simulink model "ECU_X_Enumerated_Error_Code_Generator"  (R2022a)
settings: Solver=VariableStepAuto  StartTime=0.0  StopTime=100  RelTol=1e-3
(part 2 of 2)

== system ECU_X_Enumerated_Error_Code_Generator/ECU X Error Processor/If Action Subsystem3/ECU_A_Signal_Error_Flags to Error_Code_Converter/Switch Case Action Subsystem1 ==
  Action Port : ActionPort  ActionPortLabel=case [ 1 ]:
  Constant : Constant  Value=400
  Out1 : Outport  VectorParamsAs1DForOutWhenUnconnected=off
  wires:
  Constant/1 -> Out1/1

== system ECU_X_Enumerated_Error_Code_Generator/ECU X Error Processor/If Action Subsystem3/ECU_A_Signal_Error_Flags to Error_Code_Converter/Switch Case Action Subsystem10 ==
  Action Port : ActionPort  ActionPortLabel=case [ 10 ]:
  Constant : Constant  Value=409
  Out1 : Outport  VectorParamsAs1DForOutWhenUnconnected=off
  wires:
  Constant/1 -> Out1/1

== system ECU_X_Enumerated_Error_Code_Generator/ECU X Error Processor/If Action Subsystem3/ECU_A_Signal_Error_Flags to Error_Code_Converter/Switch Case Action Subsystem11 ==
  Action Port : ActionPort  ActionPortLabel=case [ 11 ]:
  Constant : Constant  Value=500
  Out1 : Outport  VectorParamsAs1DForOutWhenUnconnected=off
  wires:
  Constant/1 -> Out1/1

== system ECU_X_Enumerated_Error_Code_Generator/ECU X Error Processor/If Action Subsystem3/ECU_A_Signal_Error_Flags to Error_Code_Converter/Switch Case Action Subsystem12 ==
  Action Port : ActionPort  ActionPortLabel=case [ 12 ]:
  Constant : Constant  Value=501
  Out1 : Outport  VectorParamsAs1DForOutWhenUnconnected=off
  wires:
  Constant/1 -> Out1/1

== system ECU_X_Enumerated_Error_Code_Generator/ECU X Error Processor/If Action Subsystem3/ECU_A_Signal_Error_Flags to Error_Code_Converter/Switch Case Action Subsystem13 ==
  Action Port : ActionPort  ActionPortLabel=case [ 13 ]:
  Constant : Constant  Value=502
  Out1 : Outport  VectorParamsAs1DForOutWhenUnconnected=off
  wires:
  Constant/1 -> Out1/1

== system ECU_X_Enumerated_Error_Code_Generator/ECU X Error Processor/If Action Subsystem3/ECU_A_Signal_Error_Flags to Error_Code_Converter/Switch Case Action Subsystem14 ==
  Action Port : ActionPort  ActionPortLabel=case [ 14 ]:
  Constant : Constant  Value=503
  Out1 : Outport  VectorParamsAs1DForOutWhenUnconnected=off
  wires:
  Constant/1 -> Out1/1

== system ECU_X_Enumerated_Error_Code_Generator/ECU X Error Processor/If Action Subsystem3/ECU_A_Signal_Error_Flags to Error_Code_Converter/Switch Case Action Subsystem15 ==
  Action Port : ActionPort  ActionPortLabel=case [ 17 ]:
  Constant : Constant  Value=506
  Out1 : Outport  VectorParamsAs1DForOutWhenUnconnected=off
  wires:
  Constant/1 -> Out1/1

== system ECU_X_Enumerated_Error_Code_Generator/ECU X Error Processor/If Action Subsystem3/ECU_A_Signal_Error_Flags to Error_Code_Converter/Switch Case Action Subsystem16 ==
  Action Port : ActionPort  ActionPortLabel=case [ 15 ]:
  Constant : Constant  Value=504
  Out1 : Outport  VectorParamsAs1DForOutWhenUnconnected=off
  wires:
  Constant/1 -> Out1/1

== system ECU_X_Enumerated_Error_Code_Generator/ECU X Error Processor/If Action Subsystem3/ECU_A_Signal_Error_Flags to Error_Code_Converter/Switch Case Action Subsystem17 ==
  Action Port : ActionPort  ActionPortLabel=case [ 16 ]:
  Constant : Constant  Value=505
  Out1 : Outport  VectorParamsAs1DForOutWhenUnconnected=off
  wires:
  Constant/1 -> Out1/1

== system ECU_X_Enumerated_Error_Code_Generator/ECU X Error Processor/If Action Subsystem3/ECU_A_Signal_Error_Flags to Error_Code_Converter/Switch Case Action Subsystem18 ==
  Action Port : ActionPort  ActionPortLabel=case [ 18 ]:
  Constant : Constant  Value=507
  Out1 : Outport  VectorParamsAs1DForOutWhenUnconnected=off
  wires:
  Constant/1 -> Out1/1

== system ECU_X_Enumerated_Error_Code_Generator/ECU X Error Processor/If Action Subsystem3/ECU_A_Signal_Error_Flags to Error_Code_Converter/Switch Case Action Subsystem19 ==
  Action Port : ActionPort  ActionPortLabel=case [ 19 ]:
  Constant : Constant  Value=508
  Out1 : Outport  VectorParamsAs1DForOutWhenUnconnected=off
  wires:
  Constant/1 -> Out1/1

== system ECU_X_Enumerated_Error_Code_Generator/ECU X Error Processor/If Action Subsystem3/ECU_A_Signal_Error_Flags to Error_Code_Converter/Switch Case Action Subsystem2 ==
  Action Port : ActionPort  ActionPortLabel=case [ 2 ]:
  Constant : Constant  Value=401
  Out1 : Outport  VectorParamsAs1DForOutWhenUnconnected=off
  wires:
  Constant/1 -> Out1/1

== system ECU_X_Enumerated_Error_Code_Generator/ECU X Error Processor/If Action Subsystem3/ECU_A_Signal_Error_Flags to Error_Code_Converter/Switch Case Action Subsystem20 ==
  Action Port : ActionPort  ActionPortLabel=case [ 20 ]:
  Constant : Constant  Value=509
  Out1 : Outport  VectorParamsAs1DForOutWhenUnconnected=off
  wires:
  Constant/1 -> Out1/1

== system ECU_X_Enumerated_Error_Code_Generator/ECU X Error Processor/If Action Subsystem3/ECU_A_Signal_Error_Flags to Error_Code_Converter/Switch Case Action Subsystem3 ==
  Action Port : ActionPort  ActionPortLabel=case [ 7 ]:
  Constant : Constant  Value=406
  Out1 : Outport  VectorParamsAs1DForOutWhenUnconnected=off
  wires:
  Constant/1 -> Out1/1

== system ECU_X_Enumerated_Error_Code_Generator/ECU X Error Processor/If Action Subsystem3/ECU_A_Signal_Error_Flags to Error_Code_Converter/Switch Case Action Subsystem4 ==
  Action Port : ActionPort  ActionPortLabel=case [ 3 ]:
  Constant : Constant  Value=402
  Out1 : Outport  VectorParamsAs1DForOutWhenUnconnected=off
  wires:
  Constant/1 -> Out1/1

== system ECU_X_Enumerated_Error_Code_Generator/ECU X Error Processor/If Action Subsystem3/ECU_A_Signal_Error_Flags to Error_Code_Converter/Switch Case Action Subsystem5 ==
  Action Port : ActionPort  ActionPortLabel=case [ 4 ]:
  Constant : Constant  Value=403
  Out1 : Outport  VectorParamsAs1DForOutWhenUnconnected=off
  wires:
  Constant/1 -> Out1/1

== system ECU_X_Enumerated_Error_Code_Generator/ECU X Error Processor/If Action Subsystem3/ECU_A_Signal_Error_Flags to Error_Code_Converter/Switch Case Action Subsystem6 ==
  Action Port : ActionPort  ActionPortLabel=case [ 5 ]:
  Constant : Constant  Value=404
  Out1 : Outport  VectorParamsAs1DForOutWhenUnconnected=off
  wires:
  Constant/1 -> Out1/1

== system ECU_X_Enumerated_Error_Code_Generator/ECU X Error Processor/If Action Subsystem3/ECU_A_Signal_Error_Flags to Error_Code_Converter/Switch Case Action Subsystem7 ==
  Action Port : ActionPort  ActionPortLabel=case [ 6 ]:
  Constant : Constant  Value=405
  Out1 : Outport  VectorParamsAs1DForOutWhenUnconnected=off
  wires:
  Constant/1 -> Out1/1

== system ECU_X_Enumerated_Error_Code_Generator/ECU X Error Processor/If Action Subsystem3/ECU_A_Signal_Error_Flags to Error_Code_Converter/Switch Case Action Subsystem8 ==
  Action Port : ActionPort  ActionPortLabel=case [ 8 ]:
  Constant : Constant  Value=407
  Out1 : Outport  VectorParamsAs1DForOutWhenUnconnected=off
  wires:
  Constant/1 -> Out1/1

== system ECU_X_Enumerated_Error_Code_Generator/ECU X Error Processor/If Action Subsystem3/ECU_A_Signal_Error_Flags to Error_Code_Converter/Switch Case Action Subsystem9 ==
  Action Port : ActionPort  ActionPortLabel=case [ 9 ]:
  Constant : Constant  Value=408
  Out1 : Outport  VectorParamsAs1DForOutWhenUnconnected=off
  wires:
  Constant/1 -> Out1/1

== system ECU_X_Enumerated_Error_Code_Generator/ECU X Error Processor/If Action Subsystem4/ECU_A_Delta_Error_Flags to Error_Code_Converter/Switch Case Action Subsystem1 ==
  Action Port : ActionPort  ActionPortLabel=case [ 1 ]:
  Constant : Constant  Value=600
  Out1 : Outport  VectorParamsAs1DForOutWhenUnconnected=off
  wires:
  Constant/1 -> Out1/1

== system ECU_X_Enumerated_Error_Code_Generator/ECU X Error Processor/If Action Subsystem4/ECU_A_Delta_Error_Flags to Error_Code_Converter/Switch Case Action Subsystem10 ==
  Action Port : ActionPort  ActionPortLabel=case [ 10 ]:
  Constant : Constant  Value=609
  Out1 : Outport  VectorParamsAs1DForOutWhenUnconnected=off
  wires:
  Constant/1 -> Out1/1

== system ECU_X_Enumerated_Error_Code_Generator/ECU X Error Processor/If Action Subsystem4/ECU_A_Delta_Error_Flags to Error_Code_Converter/Switch Case Action Subsystem11 ==
  Action Port : ActionPort  ActionPortLabel=case [ 11 ]:
  Constant : Constant  Value=610
  Out1 : Outport  VectorParamsAs1DForOutWhenUnconnected=off
  wires:
  Constant/1 -> Out1/1

== system ECU_X_Enumerated_Error_Code_Generator/ECU X Error Processor/If Action Subsystem4/ECU_A_Delta_Error_Flags to Error_Code_Converter/Switch Case Action Subsystem12 ==
  Action Port : ActionPort  ActionPortLabel=case [ 12 ]:
  Constant : Constant  Value=611
  Out1 : Outport  VectorParamsAs1DForOutWhenUnconnected=off
  wires:
  Constant/1 -> Out1/1

== system ECU_X_Enumerated_Error_Code_Generator/ECU X Error Processor/If Action Subsystem4/ECU_A_Delta_Error_Flags to Error_Code_Converter/Switch Case Action Subsystem13 ==
  Action Port : ActionPort  ActionPortLabel=case [ 13 ]:
  Constant : Constant  Value=612
  Out1 : Outport  VectorParamsAs1DForOutWhenUnconnected=off
  wires:
  Constant/1 -> Out1/1

== system ECU_X_Enumerated_Error_Code_Generator/ECU X Error Processor/If Action Subsystem4/ECU_A_Delta_Error_Flags to Error_Code_Converter/Switch Case Action Subsystem14 ==
  Action Port : ActionPort  ActionPortLabel=case [ 14 ]:
  Constant : Constant  Value=613
  Out1 : Outport  VectorParamsAs1DForOutWhenUnconnected=off
  wires:
  Constant/1 -> Out1/1

== system ECU_X_Enumerated_Error_Code_Generator/ECU X Error Processor/If Action Subsystem4/ECU_A_Delta_Error_Flags to Error_Code_Converter/Switch Case Action Subsystem15 ==
  Action Port : ActionPort  ActionPortLabel=case [ 17 ]:
  Constant : Constant  Value=700
  Out1 : Outport  VectorParamsAs1DForOutWhenUnconnected=off
  wires:
  Constant/1 -> Out1/1

== system ECU_X_Enumerated_Error_Code_Generator/ECU X Error Processor/If Action Subsystem4/ECU_A_Delta_Error_Flags to Error_Code_Converter/Switch Case Action Subsystem16 ==
  Action Port : ActionPort  ActionPortLabel=case [ 15 ]:
  Constant : Constant  Value=614
  Out1 : Outport  VectorParamsAs1DForOutWhenUnconnected=off
  wires:
  Constant/1 -> Out1/1

== system ECU_X_Enumerated_Error_Code_Generator/ECU X Error Processor/If Action Subsystem4/ECU_A_Delta_Error_Flags to Error_Code_Converter/Switch Case Action Subsystem17 ==
  Action Port : ActionPort  ActionPortLabel=case [ 16 ]:
  Constant : Constant  Value=615
  Out1 : Outport  VectorParamsAs1DForOutWhenUnconnected=off
  wires:
  Constant/1 -> Out1/1

== system ECU_X_Enumerated_Error_Code_Generator/ECU X Error Processor/If Action Subsystem4/ECU_A_Delta_Error_Flags to Error_Code_Converter/Switch Case Action Subsystem18 ==
  Action Port : ActionPort  ActionPortLabel=case [ 18 ]:
  Constant : Constant  Value=701
  Out1 : Outport  VectorParamsAs1DForOutWhenUnconnected=off
  wires:
  Constant/1 -> Out1/1

== system ECU_X_Enumerated_Error_Code_Generator/ECU X Error Processor/If Action Subsystem4/ECU_A_Delta_Error_Flags to Error_Code_Converter/Switch Case Action Subsystem19 ==
  Action Port : ActionPort  ActionPortLabel=case [ 19 ]:
  Constant : Constant  Value=702
  Out1 : Outport  VectorParamsAs1DForOutWhenUnconnected=off
  wires:
  Constant/1 -> Out1/1

== system ECU_X_Enumerated_Error_Code_Generator/ECU X Error Processor/If Action Subsystem4/ECU_A_Delta_Error_Flags to Error_Code_Converter/Switch Case Action Subsystem2 ==
  Action Port : ActionPort  ActionPortLabel=case [ 2 ]:
  Constant : Constant  Value=601
  Out1 : Outport  VectorParamsAs1DForOutWhenUnconnected=off
  wires:
  Constant/1 -> Out1/1

== system ECU_X_Enumerated_Error_Code_Generator/ECU X Error Processor/If Action Subsystem4/ECU_A_Delta_Error_Flags to Error_Code_Converter/Switch Case Action Subsystem20 ==
  Action Port : ActionPort  ActionPortLabel=case [ 21 ]:
  Constant : Constant  Value=704
  Out1 : Outport  VectorParamsAs1DForOutWhenUnconnected=off
  wires:
  Constant/1 -> Out1/1

== system ECU_X_Enumerated_Error_Code_Generator/ECU X Error Processor/If Action Subsystem4/ECU_A_Delta_Error_Flags to Error_Code_Converter/Switch Case Action Subsystem21 ==
  Action Port : ActionPort  ActionPortLabel=case [ 20 ]:
  Constant : Constant  Value=703
  Out1 : Outport  VectorParamsAs1DForOutWhenUnconnected=off
  wires:
  Constant/1 -> Out1/1

== system ECU_X_Enumerated_Error_Code_Generator/ECU X Error Processor/If Action Subsystem4/ECU_A_Delta_Error_Flags to Error_Code_Converter/Switch Case Action Subsystem22 ==
  Action Port : ActionPort  ActionPortLabel=case [ 22 ]:
  Constant : Constant  Value=705
  Out1 : Outport  VectorParamsAs1DForOutWhenUnconnected=off
  wires:
  Constant/1 -> Out1/1

== system ECU_X_Enumerated_Error_Code_Generator/ECU X Error Processor/If Action Subsystem4/ECU_A_Delta_Error_Flags to Error_Code_Converter/Switch Case Action Subsystem23 ==
  Action Port : ActionPort  ActionPortLabel=case [ 28 ]:
  Constant : Constant  Value=711
  Out1 : Outport  VectorParamsAs1DForOutWhenUnconnected=off
  wires:
  Constant/1 -> Out1/1

== system ECU_X_Enumerated_Error_Code_Generator/ECU X Error Processor/If Action Subsystem4/ECU_A_Delta_Error_Flags to Error_Code_Converter/Switch Case Action Subsystem24 ==
  Action Port : ActionPort  ActionPortLabel=case [ 32 ]:
  Constant : Constant  Value=715
  Out1 : Outport  VectorParamsAs1DForOutWhenUnconnected=off
  wires:
  Constant/1 -> Out1/1

== system ECU_X_Enumerated_Error_Code_Generator/ECU X Error Processor/If Action Subsystem4/ECU_A_Delta_Error_Flags to Error_Code_Converter/Switch Case Action Subsystem25 ==
  Action Port : ActionPort  ActionPortLabel=case [ 27 ]:
  Constant : Constant  Value=710
  Out1 : Outport  VectorParamsAs1DForOutWhenUnconnected=off
  wires:
  Constant/1 -> Out1/1

== system ECU_X_Enumerated_Error_Code_Generator/ECU X Error Processor/If Action Subsystem4/ECU_A_Delta_Error_Flags to Error_Code_Converter/Switch Case Action Subsystem26 ==
  Action Port : ActionPort  ActionPortLabel=case [ 26 ]:
  Constant : Constant  Value=709
  Out1 : Outport  VectorParamsAs1DForOutWhenUnconnected=off
  wires:
  Constant/1 -> Out1/1

== system ECU_X_Enumerated_Error_Code_Generator/ECU X Error Processor/If Action Subsystem4/ECU_A_Delta_Error_Flags to Error_Code_Converter/Switch Case Action Subsystem27 ==
  Action Port : ActionPort  ActionPortLabel=case [ 23 ]:
  Constant : Constant  Value=706
  Out1 : Outport  VectorParamsAs1DForOutWhenUnconnected=off
  wires:
  Constant/1 -> Out1/1

== system ECU_X_Enumerated_Error_Code_Generator/ECU X Error Processor/If Action Subsystem4/ECU_A_Delta_Error_Flags to Error_Code_Converter/Switch Case Action Subsystem28 ==
  Action Port : ActionPort  ActionPortLabel=case [ 25 ]:
  Constant : Constant  Value=708
  Out1 : Outport  VectorParamsAs1DForOutWhenUnconnected=off
  wires:
  Constant/1 -> Out1/1

== system ECU_X_Enumerated_Error_Code_Generator/ECU X Error Processor/If Action Subsystem4/ECU_A_Delta_Error_Flags to Error_Code_Converter/Switch Case Action Subsystem29 ==
  Action Port : ActionPort  ActionPortLabel=case [ 24 ]:
  Constant : Constant  Value=707
  Out1 : Outport  VectorParamsAs1DForOutWhenUnconnected=off
  wires:
  Constant/1 -> Out1/1

== system ECU_X_Enumerated_Error_Code_Generator/ECU X Error Processor/If Action Subsystem4/ECU_A_Delta_Error_Flags to Error_Code_Converter/Switch Case Action Subsystem3 ==
  Action Port : ActionPort  ActionPortLabel=case [ 7 ]:
  Constant : Constant  Value=606
  Out1 : Outport  VectorParamsAs1DForOutWhenUnconnected=off
  wires:
  Constant/1 -> Out1/1

== system ECU_X_Enumerated_Error_Code_Generator/ECU X Error Processor/If Action Subsystem4/ECU_A_Delta_Error_Flags to Error_Code_Converter/Switch Case Action Subsystem32 ==
  Action Port : ActionPort  ActionPortLabel=case [ 31 ]:
  Constant : Constant  Value=714
  Out1 : Outport  VectorParamsAs1DForOutWhenUnconnected=off
  wires:
  Constant/1 -> Out1/1

== system ECU_X_Enumerated_Error_Code_Generator/ECU X Error Processor/If Action Subsystem4/ECU_A_Delta_Error_Flags to Error_Code_Converter/Switch Case Action Subsystem33 ==
  Action Port : ActionPort  ActionPortLabel=case [ 30 ]:
  Constant : Constant  Value=713
  Out1 : Outport  VectorParamsAs1DForOutWhenUnconnected=off
  wires:
  Constant/1 -> Out1/1

== system ECU_X_Enumerated_Error_Code_Generator/ECU X Error Processor/If Action Subsystem4/ECU_A_Delta_Error_Flags to Error_Code_Converter/Switch Case Action Subsystem34 ==
  Action Port : ActionPort  ActionPortLabel=case [ 29 ]:
  Constant : Constant  Value=712
  Out1 : Outport  VectorParamsAs1DForOutWhenUnconnected=off
  wires:
  Constant/1 -> Out1/1

== system ECU_X_Enumerated_Error_Code_Generator/ECU X Error Processor/If Action Subsystem4/ECU_A_Delta_Error_Flags to Error_Code_Converter/Switch Case Action Subsystem4 ==
  Action Port : ActionPort  ActionPortLabel=case [ 3 ]:
  Constant : Constant  Value=602
  Out1 : Outport  VectorParamsAs1DForOutWhenUnconnected=off
  wires:
  Constant/1 -> Out1/1

== system ECU_X_Enumerated_Error_Code_Generator/ECU X Error Processor/If Action Subsystem4/ECU_A_Delta_Error_Flags to Error_Code_Converter/Switch Case Action Subsystem5 ==
  Action Port : ActionPort  ActionPortLabel=case [ 4 ]:
  Constant : Constant  Value=603
  Out1 : Outport  VectorParamsAs1DForOutWhenUnconnected=off
  wires:
  Constant/1 -> Out1/1

== system ECU_X_Enumerated_Error_Code_Generator/ECU X Error Processor/If Action Subsystem4/ECU_A_Delta_Error_Flags to Error_Code_Converter/Switch Case Action Subsystem6 ==
  Action Port : ActionPort  ActionPortLabel=case [ 5 ]:
  Constant : Constant  Value=604
  Out1 : Outport  VectorParamsAs1DForOutWhenUnconnected=off
  wires:
  Constant/1 -> Out1/1

== system ECU_X_Enumerated_Error_Code_Generator/ECU X Error Processor/If Action Subsystem4/ECU_A_Delta_Error_Flags to Error_Code_Converter/Switch Case Action Subsystem7 ==
  Action Port : ActionPort  ActionPortLabel=case [ 6 ]:
  Constant : Constant  Value=605
  Out1 : Outport  VectorParamsAs1DForOutWhenUnconnected=off
  wires:
  Constant/1 -> Out1/1

== system ECU_X_Enumerated_Error_Code_Generator/ECU X Error Processor/If Action Subsystem4/ECU_A_Delta_Error_Flags to Error_Code_Converter/Switch Case Action Subsystem8 ==
  Action Port : ActionPort  ActionPortLabel=case [ 8 ]:
  Constant : Constant  Value=607
  Out1 : Outport  VectorParamsAs1DForOutWhenUnconnected=off
  wires:
  Constant/1 -> Out1/1

== system ECU_X_Enumerated_Error_Code_Generator/ECU X Error Processor/If Action Subsystem4/ECU_A_Delta_Error_Flags to Error_Code_Converter/Switch Case Action Subsystem9 ==
  Action Port : ActionPort  ActionPortLabel=case [ 9 ]:
  Constant : Constant  Value=608
  Out1 : Outport  VectorParamsAs1DForOutWhenUnconnected=off
  wires:
  Constant/1 -> Out1/1
